simulink model "delay"  (R2023b)
settings: Solver=VariableStepAuto  StartTime=0.0  StopTime=1  RelTol=1e-3
libraries: simulink x1
settings Model: Creator=1234  LastModifiedBy=1234

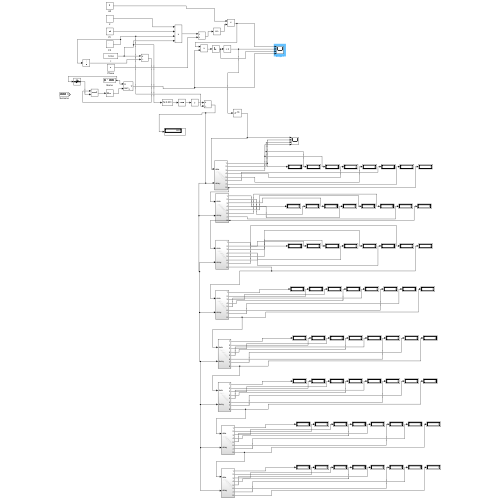
[thumbnail: Simulink's stored preview of the top-level diagram]
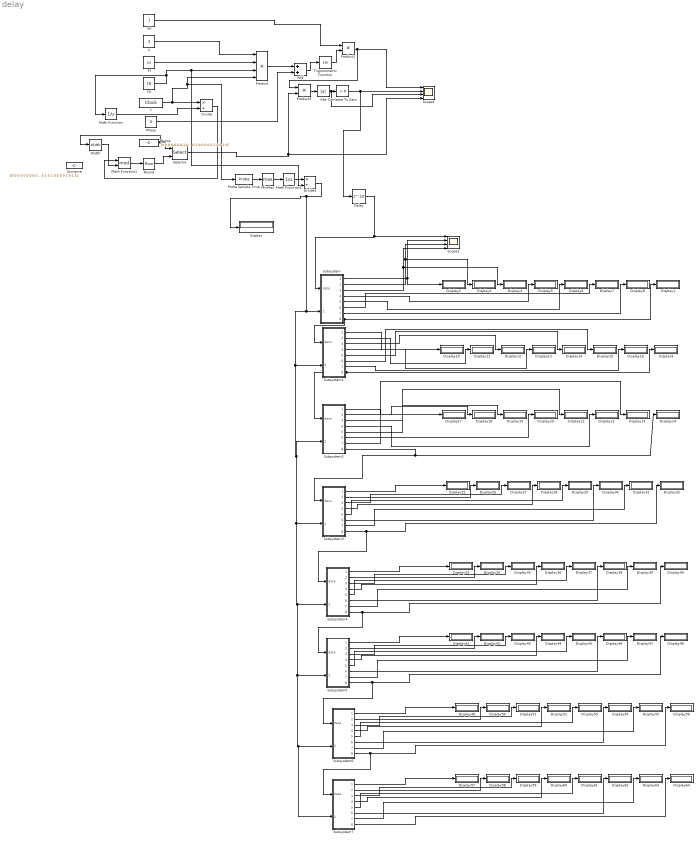
== system delay ==
  2 : Constant  Value=2
  A0 : Constant
  Abs : Abs  SaturateOnIntegerOverflow=off
  Add : Sum
  Compare To Zero : simulink/Logic and Bit Operations/Compare To Zero  relop=>  OutDataTypeStr=boolean
  Delay : Delay  DelayLength=10  InitialCondition=0
  Display{,1..64} (65 alike) : Display
  Divide : Product  Inputs=*/
  Divide1 : Product  Inputs=*/
  F0 : Constant  Value=16
  Math Function : Math  Operator=reciprocal
  Math Function1 : Math  Operator=mod
  Math Function2 : Math  Operator=reciprocal
  MinMax : MinMax  Function=max
  Name : Constant  Value=[0 0 0 0 0 0 0 1 0 0 0 0 1 1 0 0 0 0 0 0 0 1 0 1 0 0 0 1 1 0 0 0 0 0 0 0 0 0 0 1 0 0 0 0 1 1 1 0 0 0 0 0 0 1 0 0 0 0 0 1 0 0 1 0]  VectorParams1D=off
  PI : Constant  Value=pi
  Phase : Constant  Value=0
  Probe Sample Time : Probe  ProbeWidth=off  ProbeComplexSignal=off
  Product : Product  Inputs=4
  Product1 : Product
  Product2 : Product
  Round : Rounding
  Scope1 : Scope  NumInputPorts=4
  Scope2 : Scope  NumInputPorts=4
  Selector : Selector  IndexMode=Zero-based  InputPortWidth=64  IndexOptions=Index vector (port)  Indices=[1 3]  OutputSizes=1
  Subsystem : Subsystem
  Subsystem1 : Subsystem
  Subsystem2 : Subsystem
  Subsystem3 : Subsystem
  Subsystem4 : Subsystem
  Subsystem5 : Subsystem
  Subsystem6 : Subsystem
  Subsystem7 : Subsystem
  Surname : Constant  Value=[0 0 0 1 0 0 0 0 0 0 0 0 1 1 1 1 0 0 0 0 0 1 1 1 0 0 0 1 0 0 1 0 0 0 0 0 0 1 0 1 0 0 0 0 0 0 1 0 0 0 0 0 1 1 1 0 0 0 0 1 1 0 0 1 0 0 0 1 0 1 0 1 0 0 0 0 1 0 1 1]
  Trigonometric Function : Trigonometry
  Width : Width
  t : DigitalClock  SampleTime=1/1000
  wires:
  2/1 -> Product/1
  PI/1 -> Product/2
  t/1 -> Probe Sample Time/1, Product/4, Divide/1
  Phase/1 -> Add/2
  Add/1 -> Trigonometric Function/1
  Trigonometric Function/1 -> Product1/2
  A0/1 -> Product1/1
  Product1/1 -> Scope1/1, Product2/1
  Selector/1 -> Product2/2, Scope1/4
  Product/1 -> Add/1
  Math Function1/1 -> Round/1
  Round/1 -> Selector/2
  Product2/1 -> Abs/1
  Divide/1 -> Math Function1/1
  Abs/1 -> Scope1/3, Compare To Zero/1
  Compare To Zero/1 -> Delay/1, Scope1/2
  Name/1 -> Width/1, Selector/1
  Width/1 -> Math Function1/2
  Math Function/1 -> Divide/2
  F0/1 -> Math Function/1, Divide1/2, Product/3
  Probe Sample Time/1 -> MinMax/1
  MinMax/1 -> Math Function2/1
  Math Function2/1 -> Divide1/1
  Subsystem/1(Out1) -> Scope2/2, Display2/1
  Subsystem/2(Out2) -> Display3/1, Scope2/3
  Subsystem/3(Out4) -> Scope2/4, Display4/1
  Subsystem/4(Out3) -> Display5/1
  Subsystem/5(Out5) -> Display6/1
  Subsystem/6(Out6) -> Display7/1
  Subsystem/7(Out7) -> Display8/1
  Subsystem/8(Out8) -> Display1/1, Subsystem1/1(data)
  Subsystem1/1(Out1) -> Display10/1
  Subsystem1/2(Out2) -> Display11/1
  Subsystem1/3(Out4) -> Display12/1
  Subsystem1/4(Out3) -> Display13/1
  Subsystem1/5(Out5) -> Display14/1
  Subsystem1/6(Out6) -> Display15/1
  Subsystem1/7(Out7) -> Display16/1
  Subsystem1/8(Out8) -> Display9/1, Subsystem2/1(data)
  Subsystem2/1(Out1) -> Display17/1
  Subsystem2/2(Out2) -> Display18/1
  Subsystem2/3(Out4) -> Display19/1
  Subsystem2/4(Out3) -> Display20/1
  Subsystem2/5(Out5) -> Display21/1
  Subsystem2/6(Out6) -> Display22/1
  Subsystem2/7(Out7) -> Display23/1
  Subsystem2/8(Out8) -> Subsystem3/1(data), Display24/1
  Subsystem3/1(Out1) -> Display25/1
  Subsystem3/2(Out2) -> Display26/1
  Subsystem3/3(Out4) -> Display27/1
  Subsystem3/4(Out3) -> Display28/1
  Subsystem3/5(Out5) -> Display29/1
  Subsystem3/6(Out6) -> Display30/1
  Subsystem3/7(Out7) -> Display31/1
  Delay/1 -> Scope2/1, Subsystem/1(data)
  Subsystem4/3(Out4) -> Display35/1
  Subsystem4/6(Out6) -> Display38/1
  Subsystem4/2(Out2) -> Display34/1
  Subsystem4/5(Out5) -> Display37/1
  Subsystem4/7(Out7) -> Display39/1
  Subsystem4/1(Out1) -> Display33/1
  Subsystem4/4(Out3) -> Display36/1
  Subsystem3/8(Out8) -> Subsystem4/1(data), Display32/1
  Subsystem5/3(Out4) -> Display43/1
  Subsystem5/6(Out6) -> Display46/1
  Subsystem5/2(Out2) -> Display42/1
  Subsystem5/5(Out5) -> Display45/1
  Subsystem5/7(Out7) -> Display47/1
  Subsystem5/1(Out1) -> Display41/1
  Subsystem5/4(Out3) -> Display44/1
  Subsystem4/8(Out8) -> Subsystem5/1(data), Display40/1
  Subsystem6/3(Out4) -> Display51/1
  Subsystem6/6(Out6) -> Display54/1
  Subsystem6/2(Out2) -> Display50/1
  Subsystem6/5(Out5) -> Display53/1
  Subsystem6/7(Out7) -> Display55/1
  Subsystem6/1(Out1) -> Display49/1
  Subsystem6/4(Out3) -> Display52/1
  Subsystem5/8(Out8) -> Subsystem6/1(data), Display48/1
  Subsystem7/3(Out4) -> Display59/1
  Subsystem7/6(Out6) -> Display62/1
  Subsystem7/2(Out2) -> Display58/1
  Subsystem7/5(Out5) -> Display61/1
  Subsystem7/7(Out7) -> Display63/1
  Subsystem7/1(Out1) -> Display57/1
  Divide1/1 -> Subsystem7/2(delay), Subsystem6/2(delay), Subsystem5/2(delay), Subsystem4/2(delay), Subsystem3/2(delay), Subsystem2/2(delay), Subsystem1/2(delay), Subsystem/2(delay), Display/1
  Subsystem7/4(Out3) -> Display60/1
  Subsystem6/8(Out8) -> Subsystem7/1(data), Display56/1
  Subsystem7/8(Out8) -> Display64/1

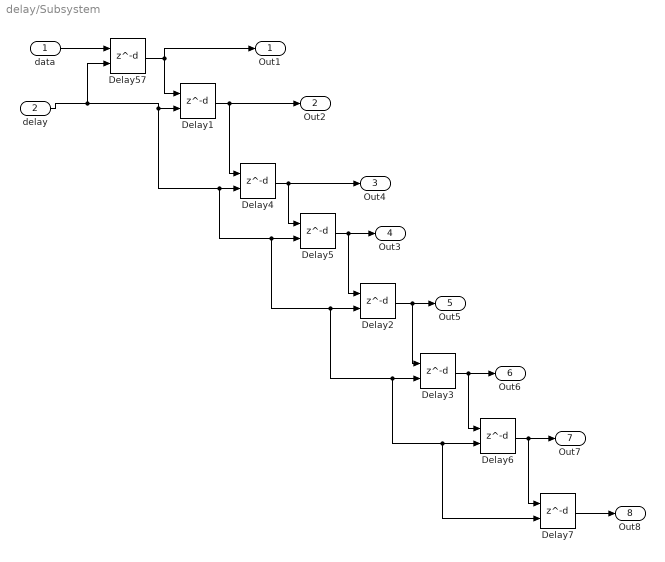
== system delay/Subsystem ==
  data : Inport
  delay : Inport  Port=2
  Delay{1..7,57} (8 alike) : Delay  DelayLengthSource=Input port  DelayLength=1  DelayLengthUpperLimit=2000  InitialCondition=0
      settings: InputPortMap=u0,p1
  Out1 : Outport
  Out2 : Outport  Port=2
  Out4 : Outport  Port=3
  Out3 : Outport  Port=4
  Out5 : Outport  Port=5
  Out6 : Outport  Port=6
  Out7 : Outport  Port=7
  Out8 : Outport  Port=8
  wires:
  Delay57/1 -> Out1/1, Delay1/1
  Delay1/1 -> Delay4/1, Out2/1
  Delay4/1 -> Delay5/1, Out4/1
  Delay5/1 -> Delay2/1, Out3/1
  Delay2/1 -> Delay3/1, Out5/1
  Delay3/1 -> Delay6/1, Out6/1
  Delay6/1 -> Delay7/1, Out7/1
  Delay7/1 -> Out8/1
  data/1 -> Delay57/1
  delay/1 -> Delay7/2, Delay6/2, Delay3/2, Delay2/2, Delay5/2, Delay4/2, Delay1/2, Delay57/2

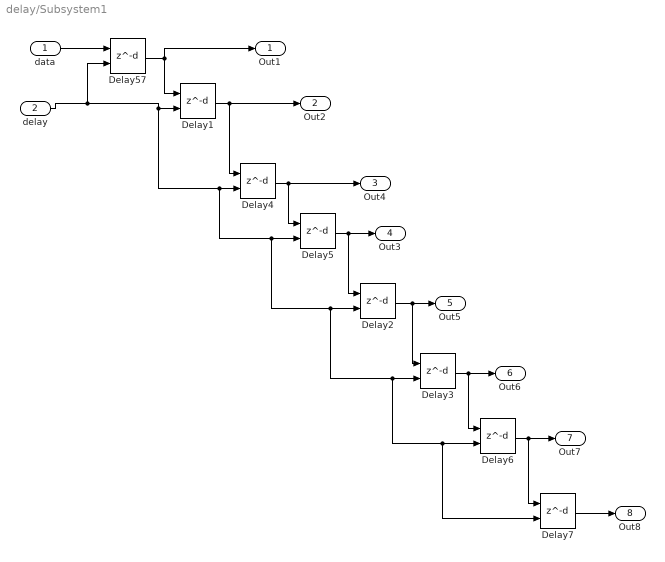
== system delay/Subsystem1 ==
  data : Inport
  delay : Inport  Port=2
  Delay{1..7,57} (8 alike) : Delay  DelayLengthSource=Input port  DelayLength=1  DelayLengthUpperLimit=2000  InitialCondition=0
      settings: InputPortMap=u0,p1
  Out1 : Outport
  Out2 : Outport  Port=2
  Out4 : Outport  Port=3
  Out3 : Outport  Port=4
  Out5 : Outport  Port=5
  Out6 : Outport  Port=6
  Out7 : Outport  Port=7
  Out8 : Outport  Port=8
  wires:
  Delay57/1 -> Out1/1, Delay1/1
  Delay1/1 -> Delay4/1, Out2/1
  Delay4/1 -> Delay5/1, Out4/1
  Delay5/1 -> Delay2/1, Out3/1
  Delay2/1 -> Delay3/1, Out5/1
  Delay3/1 -> Delay6/1, Out6/1
  Delay6/1 -> Delay7/1, Out7/1
  Delay7/1 -> Out8/1
  data/1 -> Delay57/1
  delay/1 -> Delay7/2, Delay6/2, Delay3/2, Delay2/2, Delay5/2, Delay4/2, Delay1/2, Delay57/2

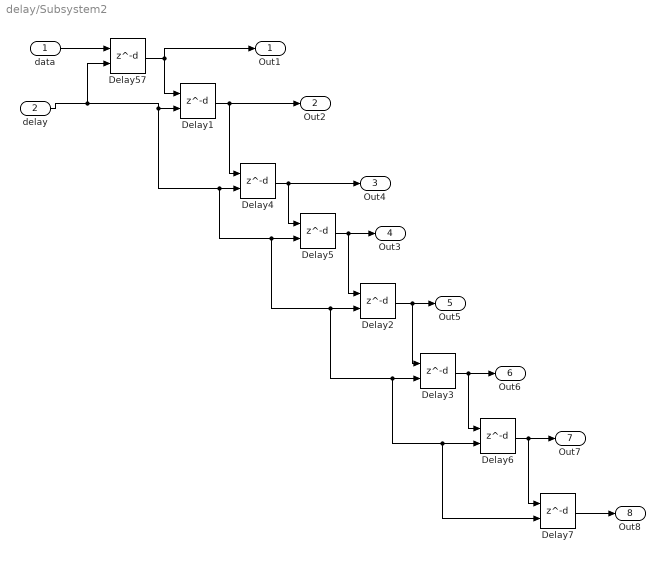
== system delay/Subsystem2 ==
  data : Inport
  delay : Inport  Port=2
  Delay{1..7,57} (8 alike) : Delay  DelayLengthSource=Input port  DelayLength=1  DelayLengthUpperLimit=2000  InitialCondition=0
      settings: InputPortMap=u0,p1
  Out1 : Outport
  Out2 : Outport  Port=2
  Out4 : Outport  Port=3
  Out3 : Outport  Port=4
  Out5 : Outport  Port=5
  Out6 : Outport  Port=6
  Out7 : Outport  Port=7
  Out8 : Outport  Port=8
  wires:
  Delay57/1 -> Out1/1, Delay1/1
  Delay1/1 -> Delay4/1, Out2/1
  Delay4/1 -> Delay5/1, Out4/1
  Delay5/1 -> Delay2/1, Out3/1
  Delay2/1 -> Delay3/1, Out5/1
  Delay3/1 -> Delay6/1, Out6/1
  Delay6/1 -> Delay7/1, Out7/1
  Delay7/1 -> Out8/1
  data/1 -> Delay57/1
  delay/1 -> Delay7/2, Delay6/2, Delay3/2, Delay2/2, Delay5/2, Delay4/2, Delay1/2, Delay57/2

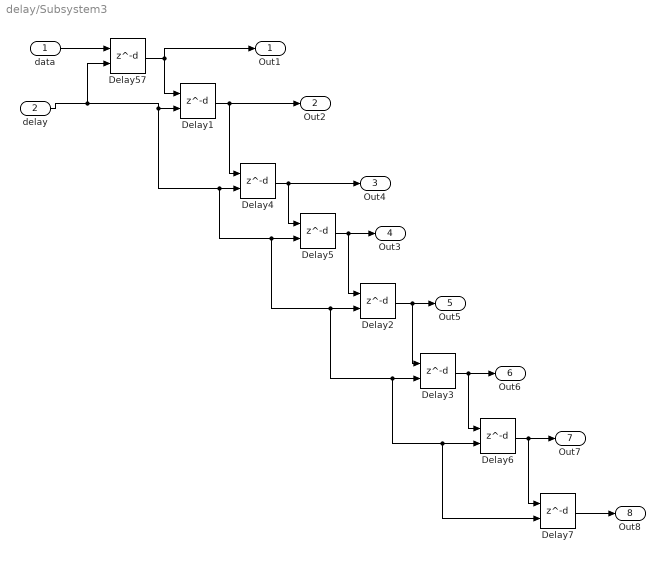
== system delay/Subsystem3 ==
  data : Inport
  delay : Inport  Port=2
  Delay{1..7,57} (8 alike) : Delay  DelayLengthSource=Input port  DelayLength=1  DelayLengthUpperLimit=2000  InitialCondition=0
      settings: InputPortMap=u0,p1
  Out1 : Outport
  Out2 : Outport  Port=2
  Out4 : Outport  Port=3
  Out3 : Outport  Port=4
  Out5 : Outport  Port=5
  Out6 : Outport  Port=6
  Out7 : Outport  Port=7
  Out8 : Outport  Port=8
  wires:
  Delay57/1 -> Out1/1, Delay1/1
  Delay1/1 -> Delay4/1, Out2/1
  Delay4/1 -> Delay5/1, Out4/1
  Delay5/1 -> Delay2/1, Out3/1
  Delay2/1 -> Delay3/1, Out5/1
  Delay3/1 -> Delay6/1, Out6/1
  Delay6/1 -> Delay7/1, Out7/1
  Delay7/1 -> Out8/1
  data/1 -> Delay57/1
  delay/1 -> Delay7/2, Delay6/2, Delay3/2, Delay2/2, Delay5/2, Delay4/2, Delay1/2, Delay57/2

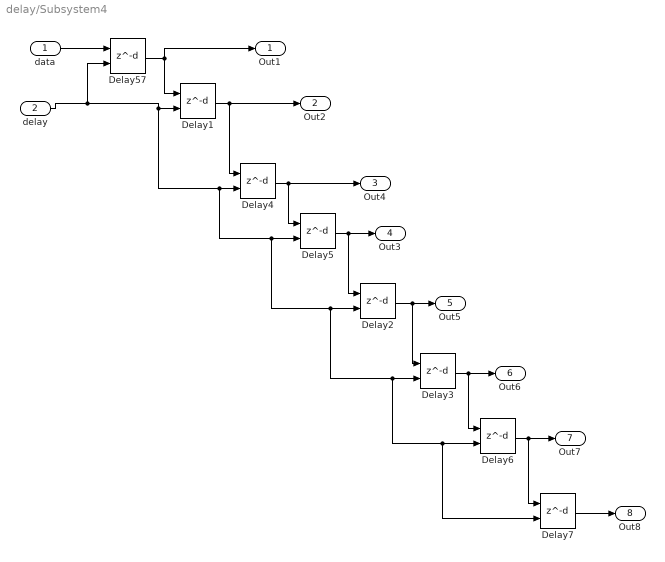
== system delay/Subsystem4 ==
  data : Inport
  delay : Inport  Port=2
  Delay{1..7,57} (8 alike) : Delay  DelayLengthSource=Input port  DelayLength=1  DelayLengthUpperLimit=2000  InitialCondition=0
      settings: InputPortMap=u0,p1
  Out1 : Outport
  Out2 : Outport  Port=2
  Out4 : Outport  Port=3
  Out3 : Outport  Port=4
  Out5 : Outport  Port=5
  Out6 : Outport  Port=6
  Out7 : Outport  Port=7
  Out8 : Outport  Port=8
  wires:
  Delay57/1 -> Out1/1, Delay1/1
  Delay1/1 -> Delay4/1, Out2/1
  Delay4/1 -> Delay5/1, Out4/1
  Delay5/1 -> Delay2/1, Out3/1
  Delay2/1 -> Delay3/1, Out5/1
  Delay3/1 -> Delay6/1, Out6/1
  Delay6/1 -> Delay7/1, Out7/1
  Delay7/1 -> Out8/1
  data/1 -> Delay57/1
  delay/1 -> Delay7/2, Delay6/2, Delay3/2, Delay2/2, Delay5/2, Delay4/2, Delay1/2, Delay57/2

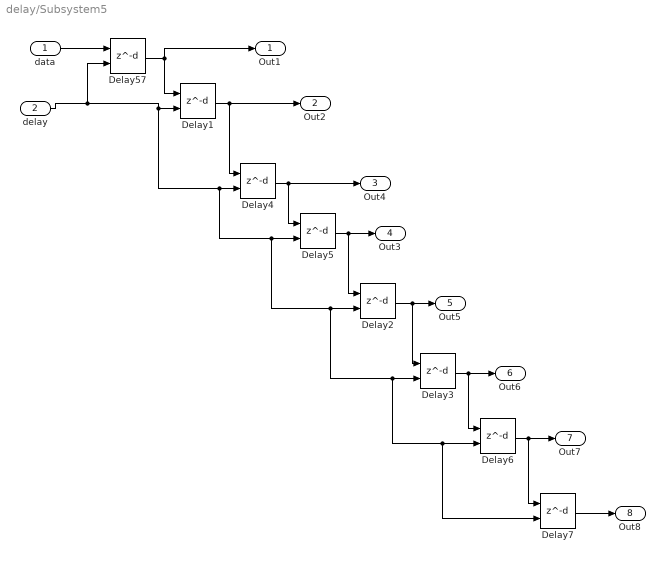
== system delay/Subsystem5 ==
  data : Inport
  delay : Inport  Port=2
  Delay{1..7,57} (8 alike) : Delay  DelayLengthSource=Input port  DelayLength=1  DelayLengthUpperLimit=2000  InitialCondition=0
      settings: InputPortMap=u0,p1
  Out1 : Outport
  Out2 : Outport  Port=2
  Out4 : Outport  Port=3
  Out3 : Outport  Port=4
  Out5 : Outport  Port=5
  Out6 : Outport  Port=6
  Out7 : Outport  Port=7
  Out8 : Outport  Port=8
  wires:
  Delay57/1 -> Out1/1, Delay1/1
  Delay1/1 -> Delay4/1, Out2/1
  Delay4/1 -> Delay5/1, Out4/1
  Delay5/1 -> Delay2/1, Out3/1
  Delay2/1 -> Delay3/1, Out5/1
  Delay3/1 -> Delay6/1, Out6/1
  Delay6/1 -> Delay7/1, Out7/1
  Delay7/1 -> Out8/1
  data/1 -> Delay57/1
  delay/1 -> Delay7/2, Delay6/2, Delay3/2, Delay2/2, Delay5/2, Delay4/2, Delay1/2, Delay57/2

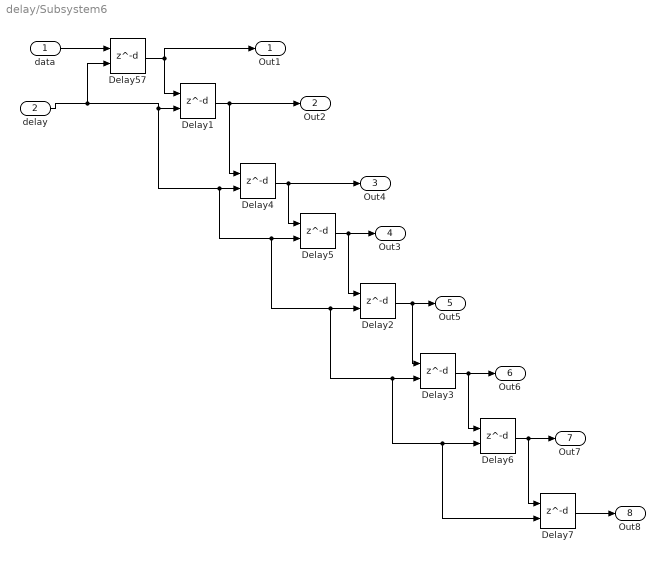
== system delay/Subsystem6 ==
  data : Inport
  delay : Inport  Port=2
  Delay{1..7,57} (8 alike) : Delay  DelayLengthSource=Input port  DelayLength=1  DelayLengthUpperLimit=2000  InitialCondition=0
      settings: InputPortMap=u0,p1
  Out1 : Outport
  Out2 : Outport  Port=2
  Out4 : Outport  Port=3
  Out3 : Outport  Port=4
  Out5 : Outport  Port=5
  Out6 : Outport  Port=6
  Out7 : Outport  Port=7
  Out8 : Outport  Port=8
  wires:
  Delay57/1 -> Out1/1, Delay1/1
  Delay1/1 -> Delay4/1, Out2/1
  Delay4/1 -> Delay5/1, Out4/1
  Delay5/1 -> Delay2/1, Out3/1
  Delay2/1 -> Delay3/1, Out5/1
  Delay3/1 -> Delay6/1, Out6/1
  Delay6/1 -> Delay7/1, Out7/1
  Delay7/1 -> Out8/1
  data/1 -> Delay57/1
  delay/1 -> Delay7/2, Delay6/2, Delay3/2, Delay2/2, Delay5/2, Delay4/2, Delay1/2, Delay57/2

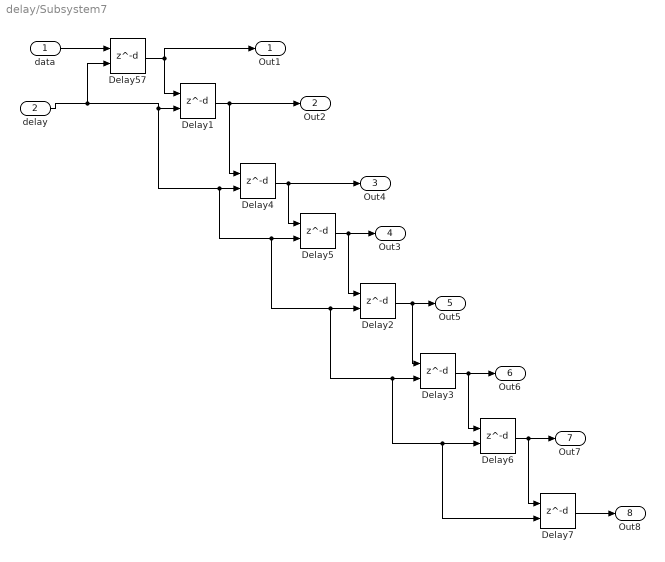
== system delay/Subsystem7 ==
  data : Inport
  delay : Inport  Port=2
  Delay{1..7,57} (8 alike) : Delay  DelayLengthSource=Input port  DelayLength=1  DelayLengthUpperLimit=2000  InitialCondition=0
      settings: InputPortMap=u0,p1
  Out1 : Outport
  Out2 : Outport  Port=2
  Out4 : Outport  Port=3
  Out3 : Outport  Port=4
  Out5 : Outport  Port=5
  Out6 : Outport  Port=6
  Out7 : Outport  Port=7
  Out8 : Outport  Port=8
  wires:
  Delay57/1 -> Out1/1, Delay1/1
  Delay1/1 -> Delay4/1, Out2/1
  Delay4/1 -> Delay5/1, Out4/1
  Delay5/1 -> Delay2/1, Out3/1
  Delay2/1 -> Delay3/1, Out5/1
  Delay3/1 -> Delay6/1, Out6/1
  Delay6/1 -> Delay7/1, Out7/1
  Delay7/1 -> Out8/1
  data/1 -> Delay57/1
  delay/1 -> Delay7/2, Delay6/2, Delay3/2, Delay2/2, Delay5/2, Delay4/2, Delay1/2, Delay57/2
